simulink model "TENSION_IZAJE"  (R2024b)
settings: Solver=VariableStepAuto  StartTime=0.0  StopTime=10.0  RelTol=1e-3
undefined symbols (not defined in the file): bwu, kwu, Lh0
settings Model: Creator=Ignacio  LastModifiedBy=juani
settings RTWCC: GPUComputeCapability=3.5

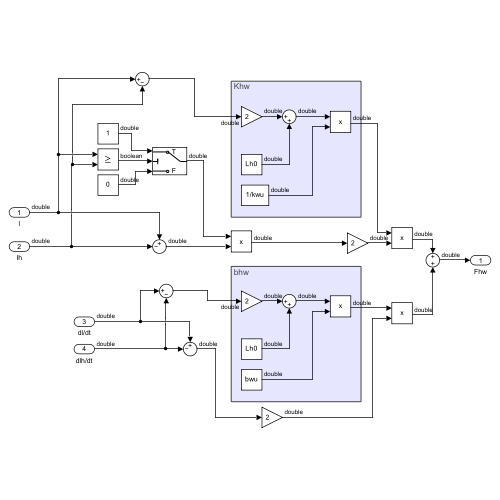
[thumbnail: Simulink's stored preview of the top-level diagram]
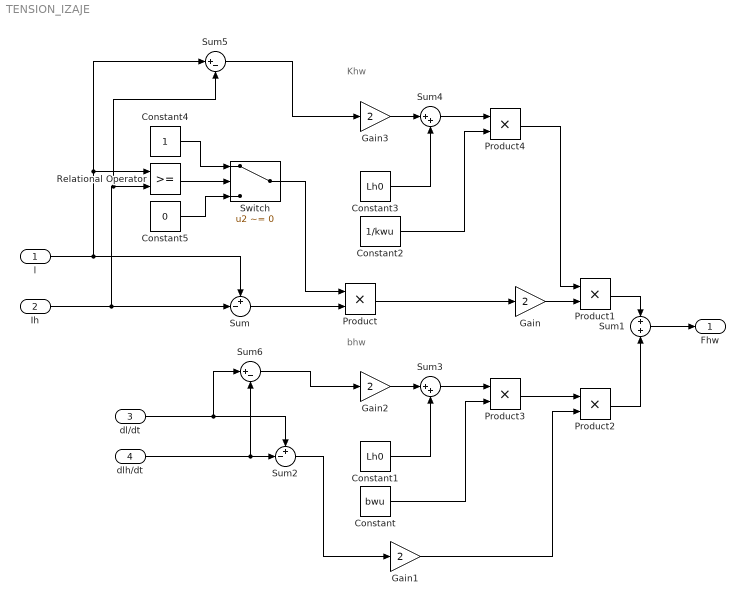
== system TENSION_IZAJE ==
  note: Khw
  note: bhw
  l : Inport
  Ih : Inport  Port=2
  dl/dt : Inport  Port=3
  dlh/dt : Inport  Port=4
  Constant : Constant  Value=bwu
  Constant1 : Constant  Value=Lh0
  Constant2 : Constant  Value=1/kwu
  Constant3 : Constant  Value=Lh0
  Constant4 : Constant  OutDataTypeStr=double
  Constant5 : Constant  Value=0  OutDataTypeStr=double
  Gain : Gain  Gain=2
  Gain1 : Gain  Gain=2
  Gain2 : Gain  Gain=2  OutDataTypeStr=Inherit: Inherit via back propagation
  Gain3 : Gain  Gain=2  OutDataTypeStr=Inherit: Inherit via back propagation
  Product{,1..4} (5 alike) : Product
  Relational Operator : RelationalOperator  OutDataTypeStr=boolean  RndMeth=Simplest  InputSameDT=off
  Sum : Sum  Inputs=+-|
  Sum1 : Sum  Inputs=+|+
  Sum2 : Sum  Inputs=+-|
  Sum3 : Sum  Inputs=|++
  Sum4 : Sum  Inputs=|++
  Sum5 : Sum  Inputs=|+-
  Sum6 : Sum  Inputs=|+-
  Switch : Switch  Criteria=u2 ~= 0  SaturateOnIntegerOverflow=off  InputSameDT=off
  Fhw : Outport
  wires:
  l/1 -> Sum/1, Sum5/1, Relational Operator/1
  Sum/1 -> Product/2
  Product/1 -> Gain/1
  Product1/1 -> Sum1/1
  dl/dt/1 -> Sum6/1, Sum2/1
  dlh/dt/1 -> Sum6/2, Sum2/2
  Sum2/1 -> Gain1/1
  Gain1/1 -> Product2/2
  Product3/1 -> Product2/1
  Product2/1 -> Sum1/2
  Sum1/1 -> Fhw/1
  Constant1/1 -> Sum3/2
  Gain2/1 -> Sum3/1
  Constant3/1 -> Sum4/2
  Gain3/1 -> Sum4/1
  Gain/1 -> Product1/2
  Product4/1 -> Product1/1
  Constant/1 -> Product3/2
  Sum3/1 -> Product3/1
  Sum4/1 -> Product4/1
  Constant2/1 -> Product4/2
  Ih/1 -> Sum/2, Sum5/2, Relational Operator/2
  Relational Operator/1 -> Switch/2
  Constant4/1 -> Switch/1
  Switch/1 -> Product/1
  Constant5/1 -> Switch/3
  Sum5/1 -> Gain3/1
  Sum6/1 -> Gain2/1
